simulink model "DiagnosisProcessor"  (R2023b)
settings: Solver=VariableStepAuto  StartTime=0.0  StopTime=10.0  RelTol=1e-3
settings Model: Creator=user  LastModifiedBy=user

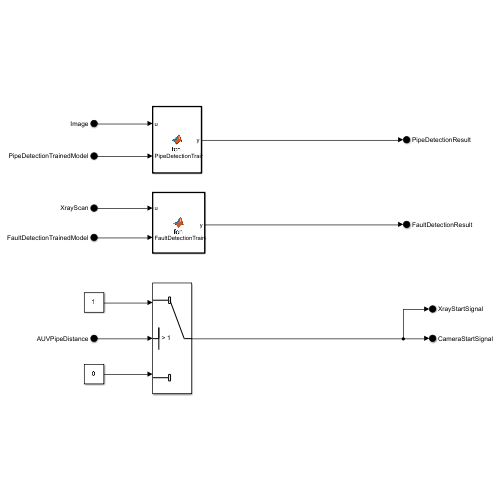
[thumbnail: Simulink's stored preview of the top-level diagram]
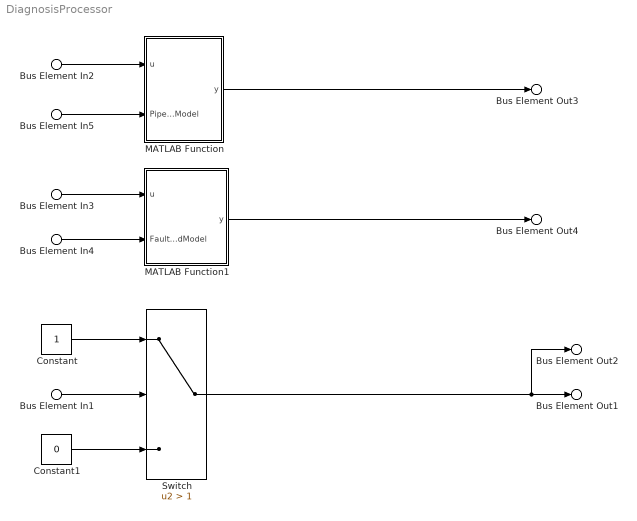
== system DiagnosisProcessor ==
  Bus Element In2 : Inport  PortName=Image
  Bus Element In4 : Inport  Port=2  PortName=FaultDetectionTrainedModel
  Bus Element In5 : Inport  Port=3  PortName=PipeDetectionTrainedModel
  Bus Element In3 : Inport  Port=4  PortName=XrayScan
  Bus Element In1 : Inport  Port=5  PortName=AUVPipeDistance
  Constant : Constant
  Constant1 : Constant  Value=0
  MATLAB Function : MATLAB Function  TreatAsAtomicUnit=on
  MATLAB Function1 : MATLAB Function  TreatAsAtomicUnit=on
  Switch : Switch  Criteria=u2 > Threshold  Threshold=1  SaturateOnIntegerOverflow=off  InputSameDT=off
  Bus Element Out1 : Outport  PortName=CameraStartSignal
  Bus Element Out2 : Outport  Port=2  PortName=XrayStartSignal
  Bus Element Out3 : Outport  Port=3  PortName=PipeDetectionResult
  Bus Element Out4 : Outport  Port=4  PortName=FaultDetectionResult
  wires:
  Bus Element In2/1 -> MATLAB Function/1(u)
  Bus Element In5/1 -> MATLAB Function/2(PipeDetectionTrainedModel)
  Bus Element In3/1 -> MATLAB Function1/1(u)
  Bus Element In4/1 -> MATLAB Function1/2(FaultDetectionTrainedModel)
  Constant/1 -> Switch/1
  Bus Element In1/1 -> Switch/2
  Constant1/1 -> Switch/3
  Switch/1 -> Bus Element Out2/1, Bus Element Out1/1
  MATLAB Function/1(y) -> Bus Element Out3/1
  MATLAB Function1/1(y) -> Bus Element Out4/1

== matlab function DiagnosisProcessor/MATLAB Function ==
  data: u input; y output; PipeDetectionTrainedModel input
function y = fcn(u, PipeDetectionTrainedModel)

u = rand(1);
if u>0.5
    y = 1;
else
    y = 0;
end

== matlab function DiagnosisProcessor/MATLAB Function1 ==
  data: u input; y output; FaultDetectionTrainedModel input
function y = fcn(u, FaultDetectionTrainedModel)

u = rand(1);
if u>0.5
    y = 1;
else
    y = 0;
end




y = u;
